simulink model "FixAngles"  (R2023a)
settings: Solver=VariableStepAuto  StartTime=0.0  StopTime=10.0  RelTol=1e-3
settings Model: Creator=yafhers  LastModifiedBy=yafhers

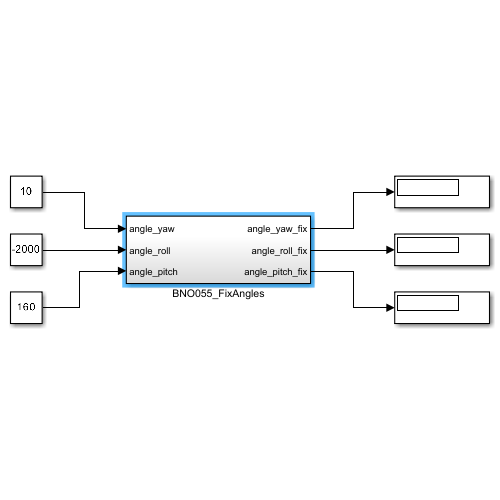
[thumbnail: Simulink's stored preview of the top-level diagram]
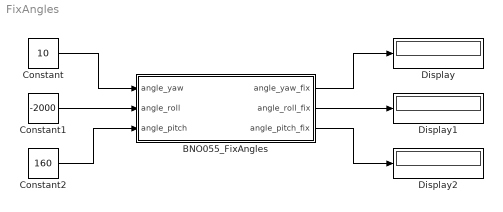
== system FixAngles ==
  BNO055_FixAngles : Subsystem
  Constant : Constant  Value=10  OutDataTypeStr=int16
  Constant1 : Constant  Value=-2000  OutDataTypeStr=int16
  Constant2 : Constant  Value=160  OutDataTypeStr=int16
  Display : Display
  Display1 : Display
  Display2 : Display
  wires:
  Constant2/1 -> BNO055_FixAngles/3(angle_pitch)
  Constant1/1 -> BNO055_FixAngles/2(angle_roll)
  Constant/1 -> BNO055_FixAngles/1(angle_yaw)
  BNO055_FixAngles/2(angle_roll_fix) -> Display1/1
  BNO055_FixAngles/1(angle_yaw_fix) -> Display/1
  BNO055_FixAngles/3(angle_pitch_fix) -> Display2/1

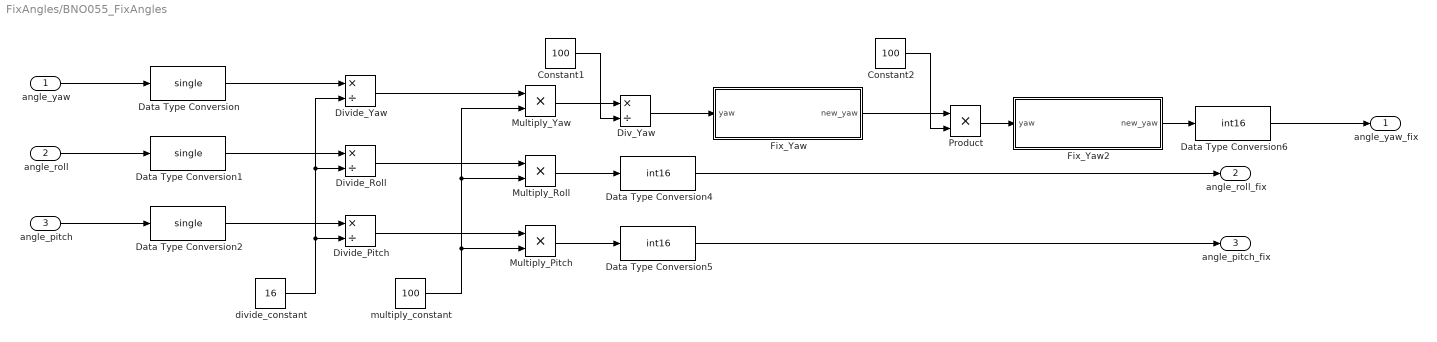
== system FixAngles/BNO055_FixAngles ==
  angle_yaw : Inport  OutDataTypeStr=int16
  angle_roll : Inport  Port=2  OutDataTypeStr=int16
  angle_pitch : Inport  Port=3  OutDataTypeStr=int16
  Constant1 : Constant  Value=100  OutDataTypeStr=single
  Constant2 : Constant  Value=100  OutDataTypeStr=single
  Data Type Conversion : DataTypeConversion  OutDataTypeStr=single  SaturateOnIntegerOverflow=off  RndMeth=Floor
  Data Type Conversion1 : DataTypeConversion  OutDataTypeStr=single  SaturateOnIntegerOverflow=off  RndMeth=Floor
  Data Type Conversion2 : DataTypeConversion  OutDataTypeStr=single  SaturateOnIntegerOverflow=off  RndMeth=Floor
  Data Type Conversion4 : DataTypeConversion  OutDataTypeStr=int16  SaturateOnIntegerOverflow=off  RndMeth=Floor
  Data Type Conversion5 : DataTypeConversion  OutDataTypeStr=int16  SaturateOnIntegerOverflow=off  RndMeth=Floor
  Data Type Conversion6 : DataTypeConversion  OutDataTypeStr=int16  SaturateOnIntegerOverflow=off  RndMeth=Floor
  Div_Yaw : Product  Inputs=*/  OutDataTypeStr=single
  Divide_Pitch : Product  Inputs=*/  OutDataTypeStr=single
  Divide_Roll : Product  Inputs=*/  OutDataTypeStr=single
  Divide_Yaw : Product  Inputs=*/  OutDataTypeStr=single
  Fix_Yaw : MATLAB Function  TreatAsAtomicUnit=on
  Fix_Yaw2 : MATLAB Function  TreatAsAtomicUnit=on
  Multiply_Pitch : Product  OutDataTypeStr=single
  Multiply_Roll : Product  OutDataTypeStr=single
  Multiply_Yaw : Product  OutDataTypeStr=single
  Product : Product  OutDataTypeStr=single
  divide_constant : Constant  Value=16  OutDataTypeStr=single
  multiply_constant : Constant  Value=100  OutDataTypeStr=single
  angle_yaw_fix : Outport  OutDataTypeStr=int16  VectorParamsAs1DForOutWhenUnconnected=off
  angle_roll_fix : Outport  Port=2  OutDataTypeStr=int16  VectorParamsAs1DForOutWhenUnconnected=off
  angle_pitch_fix : Outport  Port=3  OutDataTypeStr=int16  VectorParamsAs1DForOutWhenUnconnected=off
  wires:
  divide_constant/1 -> Divide_Yaw/2, Divide_Roll/2, Divide_Pitch/2
  angle_pitch/1 -> Data Type Conversion2/1
  Data Type Conversion2/1 -> Divide_Pitch/1
  angle_roll/1 -> Data Type Conversion1/1
  Data Type Conversion1/1 -> Divide_Roll/1
  angle_yaw/1 -> Data Type Conversion/1
  Data Type Conversion/1 -> Divide_Yaw/1
  Divide_Pitch/1 -> Multiply_Pitch/1
  Divide_Roll/1 -> Multiply_Roll/1
  multiply_constant/1 -> Multiply_Pitch/2, Multiply_Roll/2, Multiply_Yaw/2
  Multiply_Pitch/1 -> Data Type Conversion5/1
  Multiply_Roll/1 -> Data Type Conversion4/1
  Data Type Conversion4/1 -> angle_roll_fix/1
  Data Type Conversion5/1 -> angle_pitch_fix/1
  Divide_Yaw/1 -> Multiply_Yaw/1
  Div_Yaw/1 -> Fix_Yaw/1(yaw)
  Constant1/1 -> Div_Yaw/2
  Constant2/1 -> Product/2
  Data Type Conversion6/1 -> angle_yaw_fix/1
  Multiply_Yaw/1 -> Div_Yaw/1
  Fix_Yaw/1(new_yaw) -> Product/1
  Fix_Yaw2/1(new_yaw) -> Data Type Conversion6/1
  Product/1 -> Fix_Yaw2/1(yaw)

== matlab function FixAngles/BNO055_FixAngles/Fix_Yaw ==
  data: yaw input; new_yaw output
function new_yaw = fix_yaw(yaw)
    if yaw < 0
        new_yaw = 685 - (yaw * (-1));
    else
        new_yaw = yaw;
    end
end

== matlab function FixAngles/BNO055_FixAngles/Fix_Yaw2 ==
  data: yaw input; new_yaw output
function new_yaw = fix_yaw(yaw)
    if yaw < 0
        new_yaw = 65000 - (yaw * (-1));
    else
        new_yaw = yaw;
    end
end
